simulink model "SWC_DID_type"  (R2021b)
settings: Solver=FixedStepDiscrete  StartTime=0.0  StopTime=10.0  RelTol=1e-3
(part 2 of 2)

== system SWC_DID_type/P_DIDWriteCDD/run_DIDSet_RUNTM_sys ==
  note: Added blocks
  note: Added blocks
  note: Added blocks
  note: Added blocks
  function : TriggerPort  TriggerType=function-call  IsSimulinkFunction=on  FunctionName=run_DIDSet_RUNTM  VariantControl=(inherit)
  Terminator_1 : Terminator
  Terminator_2 : Terminator
  Terminator_3 : Terminator
  u16_DIDNum_RUNTM : ArgIn  OutDataTypeStr=uint16  ArgumentName=u16_DIDNum_RUNTM
  u16_DIDLen_RUNTM : ArgIn  Port=2  OutDataTypeStr=uint16  ArgumentName=u16_DIDLen_RUNTM
  u8Array2_RUNTM : ArgIn  Port=3  OutDataTypeStr=uint8  PortDimensions=2  ArgumentName=u8Array2_RUNTM
  wires:
  u16_DIDNum_RUNTM/1 -> Terminator_1/1
  u16_DIDLen_RUNTM/1 -> Terminator_2/1
  u8Array2_RUNTM/1 -> Terminator_3/1

== system SWC_DID_type/P_DIDWriteCDD/run_DIDSet_SensorMode_sys ==
  function : TriggerPort  TriggerType=function-call  IsSimulinkFunction=on  FunctionName=run_DIDSet_SensorMode  VariantControl=(inherit)
  Terminator_1 : Terminator
  Terminator_2 : Terminator
  Terminator_3 : Terminator
  u16_DIDNum_SensorMode : ArgIn  OutDataTypeStr=uint16  ArgumentName=u16_DIDNum_SensorMode
  u16_DIDLen_SensorMode : ArgIn  Port=2  OutDataTypeStr=uint16  ArgumentName=u16_DIDLen_SensorMode
  u8_SensorMode : ArgIn  Port=3  OutDataTypeStr=uint8  ArgumentName=u8_SensorMode
  wires:
  u16_DIDNum_SensorMode/1 -> Terminator_1/1
  u16_DIDLen_SensorMode/1 -> Terminator_2/1
  u8_SensorMode/1 -> Terminator_3/1

== system SWC_DID_type/P_DIDWriteCDD/run_DIDSet_TPMSLearnSta_sys ==
  function : TriggerPort  TriggerType=function-call  IsSimulinkFunction=on  FunctionName=run_DIDSet_TPMSLearnSta  VariantControl=(inherit)
  Terminator_1 : Terminator
  Terminator_2 : Terminator
  Terminator_3 : Terminator
  u16_DIDNum_TPMSLearnSta : ArgIn  OutDataTypeStr=uint16  ArgumentName=u16_DIDNum_TPMSLearnSta
  u16_DIDLen_TPMSLearnSta : ArgIn  Port=2  OutDataTypeStr=uint16  ArgumentName=u16_DIDLen_TPMSLearnSta
  u8_TPMSLearnSta : ArgIn  Port=3  OutDataTypeStr=uint8  ArgumentName=u8_TPMSLearnSta
  wires:
  u16_DIDNum_TPMSLearnSta/1 -> Terminator_1/1
  u16_DIDLen_TPMSLearnSta/1 -> Terminator_2/1
  u8_TPMSLearnSta/1 -> Terminator_3/1

== system SWC_DID_type/P_DIDWriteCDD/run_DIDSet_TestGroup_sys ==
  note: Added blocks
  note: Added blocks
  note: Added blocks
  note: Added blocks
  function : TriggerPort  TriggerType=function-call  IsSimulinkFunction=on  FunctionName=run_DIDSet_TestGroup  VariantControl=(inherit)
  Terminator_1 : Terminator
  Terminator_2 : Terminator
  Terminator_3 : Terminator
  u16_DIDNum_TestGroup : ArgIn  OutDataTypeStr=uint16  ArgumentName=u16_DIDNum_TestGroup
  u16_DIDLen_TestGroup : ArgIn  Port=2  OutDataTypeStr=uint16  ArgumentName=u16_DIDLen_TestGroup
  u8Array12_TestGroup : ArgIn  Port=3  OutDataTypeStr=uint8  PortDimensions=12  ArgumentName=u8Array12_TestGroup
  wires:
  u16_DIDNum_TestGroup/1 -> Terminator_1/1
  u16_DIDLen_TestGroup/1 -> Terminator_2/1
  u8Array12_TestGroup/1 -> Terminator_3/1

== system SWC_DID_type/P_DIDWriteCDD/run_DIDSet_TireSize_sys ==
  function : TriggerPort  TriggerType=function-call  IsSimulinkFunction=on  FunctionName=run_DIDSet_TireSize  VariantControl=(inherit)
  Terminator_1 : Terminator
  Terminator_2 : Terminator
  Terminator_3 : Terminator
  u16_DIDNum_TireSize : ArgIn  OutDataTypeStr=uint16  ArgumentName=u16_DIDNum_TireSize
  u16_DIDLen_TireSize : ArgIn  Port=2  OutDataTypeStr=uint16  ArgumentName=u16_DIDLen_TireSize
  u8Array16_TireSize : ArgIn  Port=3  OutDataTypeStr=uint8  PortDimensions=16  ArgumentName=u8Array16_TireSize
  wires:
  u16_DIDNum_TireSize/1 -> Terminator_1/1
  u16_DIDLen_TireSize/1 -> Terminator_2/1
  u8Array16_TireSize/1 -> Terminator_3/1

== system SWC_DID_type/P_DIDWriteCDD/run_DIDSet_TurnLampFLThreCurr_sys ==
  note: Added blocks
  note: Added blocks
  note: Added blocks
  note: Added blocks
  function : TriggerPort  TriggerType=function-call  IsSimulinkFunction=on  FunctionName=run_DIDSet_TurnLampFLThreCurr  VariantControl=(inherit)
  Terminator_1 : Terminator
  Terminator_2 : Terminator
  Terminator_3 : Terminator
  u16_DIDNum_TurnLampFLThreCurr : ArgIn  OutDataTypeStr=uint16  ArgumentName=u16_DIDNum_TurnLampFLThreCurr
  u16_DIDLen_TurnLampFLThreCurr : ArgIn  Port=2  OutDataTypeStr=uint16  ArgumentName=u16_DIDLen_TurnLampFLThreCurr
  u8_TurnLampFLThreCurr : ArgIn  Port=3  OutDataTypeStr=uint8  ArgumentName=u8_TurnLampFLThreCurr
  wires:
  u16_DIDNum_TurnLampFLThreCurr/1 -> Terminator_1/1
  u16_DIDLen_TurnLampFLThreCurr/1 -> Terminator_2/1
  u8_TurnLampFLThreCurr/1 -> Terminator_3/1

== system SWC_DID_type/P_DIDWriteCDD/run_DIDSet_TurnLampFRThreCurr_sys ==
  note: Added blocks
  note: Added blocks
  note: Added blocks
  note: Added blocks
  function : TriggerPort  TriggerType=function-call  IsSimulinkFunction=on  FunctionName=run_DIDSet_TurnLampFRThreCurr  VariantControl=(inherit)
  Terminator_1 : Terminator
  Terminator_2 : Terminator
  Terminator_3 : Terminator
  u16_DIDNum_TurnLampFRThreCurr : ArgIn  OutDataTypeStr=uint16  ArgumentName=u16_DIDNum_TurnLampFRThreCurr
  u16_DIDLen_TurnLampFRThreCurr : ArgIn  Port=2  OutDataTypeStr=uint16  ArgumentName=u16_DIDLen_TurnLampFRThreCurr
  u8_TurnLampFRThreCurr : ArgIn  Port=3  OutDataTypeStr=uint8  ArgumentName=u8_TurnLampFRThreCurr
  wires:
  u16_DIDNum_TurnLampFRThreCurr/1 -> Terminator_1/1
  u16_DIDLen_TurnLampFRThreCurr/1 -> Terminator_2/1
  u8_TurnLampFRThreCurr/1 -> Terminator_3/1

== system SWC_DID_type/P_DIDWriteCDD/run_DIDSet_TurnLampRLThreCurr_sys ==
  note: Added blocks
  note: Added blocks
  note: Added blocks
  note: Added blocks
  function : TriggerPort  TriggerType=function-call  IsSimulinkFunction=on  FunctionName=run_DIDSet_TurnLampRLThreCurr  VariantControl=(inherit)
  Terminator_1 : Terminator
  Terminator_2 : Terminator
  Terminator_3 : Terminator
  u16_DIDNum_TurnLampRLThreCurr : ArgIn  OutDataTypeStr=uint16  ArgumentName=u16_DIDNum_TurnLampRLThreCurr
  u16_DIDLen_TurnLampRLThreCurr : ArgIn  Port=2  OutDataTypeStr=uint16  ArgumentName=u16_DIDLen_TurnLampRLThreCurr
  u8_TurnLampRLThreCurr : ArgIn  Port=3  OutDataTypeStr=uint8  ArgumentName=u8_TurnLampRLThreCurr
  wires:
  u16_DIDNum_TurnLampRLThreCurr/1 -> Terminator_1/1
  u16_DIDLen_TurnLampRLThreCurr/1 -> Terminator_2/1
  u8_TurnLampRLThreCurr/1 -> Terminator_3/1

== system SWC_DID_type/P_DIDWriteCDD/run_DIDSet_TurnLampRRThreCurr_sys ==
  note: Added blocks
  note: Added blocks
  note: Added blocks
  note: Added blocks
  function : TriggerPort  TriggerType=function-call  IsSimulinkFunction=on  FunctionName=run_DIDSet_TurnLampRRThreCurr  VariantControl=(inherit)
  Terminator_1 : Terminator
  Terminator_2 : Terminator
  Terminator_3 : Terminator
  u16_DIDNum_TurnLampRRThreCurr : ArgIn  OutDataTypeStr=uint16  ArgumentName=u16_DIDNum_TurnLampRRThreCurr
  u16_DIDLen_TurnLampRRThreCurr : ArgIn  Port=2  OutDataTypeStr=uint16  ArgumentName=u16_DIDLen_TurnLampRRThreCurr
  u8_TurnLampRRThreCurr : ArgIn  Port=3  OutDataTypeStr=uint8  ArgumentName=u8_TurnLampRRThreCurr
  wires:
  u16_DIDNum_TurnLampRRThreCurr/1 -> Terminator_1/1
  u16_DIDLen_TurnLampRRThreCurr/1 -> Terminator_2/1
  u8_TurnLampRRThreCurr/1 -> Terminator_3/1

== system SWC_DID_type/P_DIDWriteCDD/run_DIDSet_UIDSta_sys ==
  note: Added blocks
  note: Added blocks
  note: Added blocks
  note: Added blocks
  function : TriggerPort  TriggerType=function-call  IsSimulinkFunction=on  FunctionName=run_DIDSet_UIDSta  VariantControl=(inherit)
  Terminator_1 : Terminator
  Terminator_2 : Terminator
  Terminator_3 : Terminator
  u16_DIDNum_UIDSta : ArgIn  OutDataTypeStr=uint16  ArgumentName=u16_DIDNum_UIDSta
  u16_DIDLen_UIDSta : ArgIn  Port=2  OutDataTypeStr=uint16  ArgumentName=u16_DIDLen_UIDSta
  u8Array26_UIDSta : ArgIn  Port=3  OutDataTypeStr=uint8  PortDimensions=26  ArgumentName=u8Array26_UIDSta
  wires:
  u16_DIDNum_UIDSta/1 -> Terminator_1/1
  u16_DIDLen_UIDSta/1 -> Terminator_2/1
  u8Array26_UIDSta/1 -> Terminator_3/1

== system SWC_DID_type/P_DIDWriteCDD/run_DIDSet_USSConfig_sys ==
  function : TriggerPort  TriggerType=function-call  IsSimulinkFunction=on  FunctionName=run_DIDSet_USSConfig  VariantControl=(inherit)
  Terminator_1 : Terminator
  Terminator_2 : Terminator
  Terminator_3 : Terminator
  u16_DIDNum_USSConfig : ArgIn  OutDataTypeStr=uint16  ArgumentName=u16_DIDNum_USSConfig
  u16_DIDLen_USSConfig : ArgIn  Port=2  OutDataTypeStr=uint16  ArgumentName=u16_DIDLen_USSConfig
  u8Array16_USSConfig : ArgIn  Port=3  OutDataTypeStr=uint8  PortDimensions=16  ArgumentName=u8Array16_USSConfig
  wires:
  u16_DIDNum_USSConfig/1 -> Terminator_1/1
  u16_DIDLen_USSConfig/1 -> Terminator_2/1
  u8Array16_USSConfig/1 -> Terminator_3/1

== system SWC_DID_type/P_DIDWriteCDD/run_DIDSet_UWBAnchorSta_sys ==
  note: Added blocks
  note: Added blocks
  note: Added blocks
  note: Added blocks
  function : TriggerPort  TriggerType=function-call  IsSimulinkFunction=on  FunctionName=run_DIDSet_UWBAnchorSta  VariantControl=(inherit)
  Terminator_1 : Terminator
  Terminator_2 : Terminator
  Terminator_3 : Terminator
  u16_DIDNum_UWBAnchorSta : ArgIn  OutDataTypeStr=uint16  ArgumentName=u16_DIDNum_UWBAnchorSta
  u16_DIDLen_UWBAnchorSta : ArgIn  Port=2  OutDataTypeStr=uint16  ArgumentName=u16_DIDLen_UWBAnchorSta
  u8Array93_UWBAnchorSta : ArgIn  Port=3  OutDataTypeStr=uint8  PortDimensions=93  ArgumentName=u8Array93_UWBAnchorSta
  wires:
  u16_DIDNum_UWBAnchorSta/1 -> Terminator_1/1
  u16_DIDLen_UWBAnchorSta/1 -> Terminator_2/1
  u8Array93_UWBAnchorSta/1 -> Terminator_3/1

== system SWC_DID_type/P_DIDWriteCDD/run_DIDSet_VIN_sys ==
  note: Added blocks
  note: Added blocks
  note: Added blocks
  note: Added blocks
  function : TriggerPort  TriggerType=function-call  IsSimulinkFunction=on  FunctionName=run_DIDSet_VIN  VariantControl=(inherit)
  Terminator_1 : Terminator
  Terminator_2 : Terminator
  Terminator_3 : Terminator
  u16_DIDNum_VIN : ArgIn  OutDataTypeStr=uint16  ArgumentName=u16_DIDNum_VIN
  u16_DIDLen_VIN : ArgIn  Port=2  OutDataTypeStr=uint16  ArgumentName=u16_DIDLen_VIN
  u8Array17_VIN : ArgIn  Port=3  OutDataTypeStr=uint8  PortDimensions=17  ArgumentName=u8Array17_VIN
  wires:
  u16_DIDNum_VIN/1 -> Terminator_1/1
  u16_DIDLen_VIN/1 -> Terminator_2/1
  u8Array17_VIN/1 -> Terminator_3/1

== system SWC_DID_type/P_DIDWriteCDD/run_DIDSet_VSS_sys ==
  note: Added blocks
  note: Added blocks
  note: Added blocks
  note: Added blocks
  function : TriggerPort  TriggerType=function-call  IsSimulinkFunction=on  FunctionName=run_DIDSet_VSS  VariantControl=(inherit)
  Terminator_1 : Terminator
  Terminator_2 : Terminator
  Terminator_3 : Terminator
  u16_DIDNum_VSS : ArgIn  OutDataTypeStr=uint16  ArgumentName=u16_DIDNum_VSS
  u16_DIDLen_VSS : ArgIn  Port=2  OutDataTypeStr=uint16  ArgumentName=u16_DIDLen_VSS
  u8_VSS : ArgIn  Port=3  OutDataTypeStr=uint8  ArgumentName=u8_VSS
  wires:
  u16_DIDNum_VSS/1 -> Terminator_1/1
  u16_DIDLen_VSS/1 -> Terminator_2/1
  u8_VSS/1 -> Terminator_3/1

== system SWC_DID_type/P_DIDWriteCDD/run_DIDSet_WhlPres_sys ==
  function : TriggerPort  TriggerType=function-call  IsSimulinkFunction=on  FunctionName=run_DIDSet_WhlPres  VariantControl=(inherit)
  Terminator_1 : Terminator
  Terminator_2 : Terminator
  Terminator_3 : Terminator
  u16_DIDNum_WhlPres : ArgIn  OutDataTypeStr=uint16  ArgumentName=u16_DIDNum_WhlPres
  u16_DIDLen_WhlPres : ArgIn  Port=2  OutDataTypeStr=uint16  ArgumentName=u16_DIDLen_WhlPres
  u8Array4_WhlPres : ArgIn  Port=3  OutDataTypeStr=uint8  PortDimensions=4  ArgumentName=u8Array4_WhlPres
  wires:
  u16_DIDNum_WhlPres/1 -> Terminator_1/1
  u16_DIDLen_WhlPres/1 -> Terminator_2/1
  u8Array4_WhlPres/1 -> Terminator_3/1

== system SWC_DID_type/P_DIDWriteCDD/run_DIDSet_WhlSensorBattSta_sys ==
  function : TriggerPort  TriggerType=function-call  IsSimulinkFunction=on  FunctionName=run_DIDSet_WhlSensorBattSta  VariantControl=(inherit)
  Terminator_1 : Terminator
  Terminator_2 : Terminator
  Terminator_3 : Terminator
  u16_DIDNum_WhlSensorBattSta : ArgIn  OutDataTypeStr=uint16  ArgumentName=u16_DIDNum_WhlSensorBattSta
  u16_DIDLen_WhlSensorBattSta : ArgIn  Port=2  OutDataTypeStr=uint16  ArgumentName=u16_DIDLen_WhlSensorBattSta
  u8_WhlSensorBattSta : ArgIn  Port=3  OutDataTypeStr=uint8  ArgumentName=u8_WhlSensorBattSta
  wires:
  u16_DIDNum_WhlSensorBattSta/1 -> Terminator_1/1
  u16_DIDLen_WhlSensorBattSta/1 -> Terminator_2/1
  u8_WhlSensorBattSta/1 -> Terminator_3/1

== system SWC_DID_type/P_DIDWriteCDD/run_DIDSet_WhlTmp_sys ==
  function : TriggerPort  TriggerType=function-call  IsSimulinkFunction=on  FunctionName=run_DIDSet_WhlTmp  VariantControl=(inherit)
  Terminator_1 : Terminator
  Terminator_2 : Terminator
  Terminator_3 : Terminator
  u16_DIDNum_WhlTmp : ArgIn  OutDataTypeStr=uint16  ArgumentName=u16_DIDNum_WhlTmp
  u16_DIDLen_WhlTmp : ArgIn  Port=2  OutDataTypeStr=uint16  ArgumentName=u16_DIDLen_WhlTmp
  u8Array4_WhlTmp : ArgIn  Port=3  OutDataTypeStr=uint8  PortDimensions=4  ArgumentName=u8Array4_WhlTmp
  wires:
  u16_DIDNum_WhlTmp/1 -> Terminator_1/1
  u16_DIDLen_WhlTmp/1 -> Terminator_2/1
  u8Array4_WhlTmp/1 -> Terminator_3/1

== system SWC_DID_type/P_DIDWriteCDD/run_DIDSet_WipRLSCmdCutFilter_sys ==
  function : TriggerPort  TriggerType=function-call  IsSimulinkFunction=on  FunctionName=run_DIDSet_WipRLSCmdCutFilter  VariantControl=(inherit)
  Terminator_1 : Terminator
  Terminator_2 : Terminator
  Terminator_3 : Terminator
  u16_DIDNum_WipRLSCmdCutFilter : ArgIn  OutDataTypeStr=uint16  ArgumentName=u16_DIDNum_WipRLSCmdCutFilter
  u16_DIDLen_WipRLSCmdCutFilter : ArgIn  Port=2  OutDataTypeStr=uint16  ArgumentName=u16_DIDLen_WipRLSCmdCutFilter
  u8_WipRLSCmdCutFilter : ArgIn  Port=3  OutDataTypeStr=uint8  ArgumentName=u8_WipRLSCmdCutFilter
  wires:
  u16_DIDNum_WipRLSCmdCutFilter/1 -> Terminator_1/1
  u16_DIDLen_WipRLSCmdCutFilter/1 -> Terminator_2/1
  u8_WipRLSCmdCutFilter/1 -> Terminator_3/1

== system SWC_DID_type/P_DIDWriteCDD/run_DIDSet_WipRLSCmdHoldFilter_sys ==
  function : TriggerPort  TriggerType=function-call  IsSimulinkFunction=on  FunctionName=run_DIDSet_WipRLSCmdHoldFilter  VariantControl=(inherit)
  Terminator_1 : Terminator
  Terminator_2 : Terminator
  Terminator_3 : Terminator
  u16_DIDNum_WipRLSCmdHoldFilter : ArgIn  OutDataTypeStr=uint16  ArgumentName=u16_DIDNum_WipRLSCmdHoldFilter
  u16_DIDLen_WipRLSCmdHoldFilter : ArgIn  Port=2  OutDataTypeStr=uint16  ArgumentName=u16_DIDLen_WipRLSCmdHoldFilter
  u8_WipRLSCmdHoldFilter : ArgIn  Port=3  OutDataTypeStr=uint8  ArgumentName=u8_WipRLSCmdHoldFilter
  wires:
  u16_DIDNum_WipRLSCmdHoldFilter/1 -> Terminator_1/1
  u16_DIDLen_WipRLSCmdHoldFilter/1 -> Terminator_2/1
  u8_WipRLSCmdHoldFilter/1 -> Terminator_3/1

== system SWC_DID_type/P_DIDWriteCDD/run_DIDSet_XWDMode_sys ==
  function : TriggerPort  TriggerType=function-call  IsSimulinkFunction=on  FunctionName=run_DIDSet_XWDMode  VariantControl=(inherit)
  Terminator_1 : Terminator
  Terminator_2 : Terminator
  Terminator_3 : Terminator
  u16_DIDNum_XWDMode : ArgIn  OutDataTypeStr=uint16  ArgumentName=u16_DIDNum_XWDMode
  u16_DIDLen_XWDMode : ArgIn  Port=2  OutDataTypeStr=uint16  ArgumentName=u16_DIDLen_XWDMode
  u8_XWDMode : ArgIn  Port=3  OutDataTypeStr=uint8  ArgumentName=u8_XWDMode
  wires:
  u16_DIDNum_XWDMode/1 -> Terminator_1/1
  u16_DIDLen_XWDMode/1 -> Terminator_2/1
  u8_XWDMode/1 -> Terminator_3/1
